simulink model "MOTOR_GENERATOR_SYSTEM_SIMULINK"  (R2023a)
settings: Solver=ode4  StartTime=0.0  StopTime=6.0  FixedStep=StepSize  RelTol=1e-3
values from neighbouring files (symbols this model uses):
  Jg = 0.05    [MOTOR_GENERATOR_SYSTEM_SCRIPT.m]
  Jm = 0.04    [MOTOR_GENERATOR_SYSTEM_SCRIPT.m]
  kag = 0.25    [MOTOR_GENERATOR_SYSTEM_SCRIPT.m]
  kam = 0.3    [MOTOR_GENERATOR_SYSTEM_SCRIPT.m]
  kfg = 0.0008    [MOTOR_GENERATOR_SYSTEM_SCRIPT.m]
  kfm = 0.0007    [MOTOR_GENERATOR_SYSTEM_SCRIPT.m]
  Lag = 0.06    [MOTOR_GENERATOR_SYSTEM_SCRIPT.m]
  Lam = 0.05    [MOTOR_GENERATOR_SYSTEM_SCRIPT.m]
  Rag = 0.3    [MOTOR_GENERATOR_SYSTEM_SCRIPT.m]
  Ram = 0.4    [MOTOR_GENERATOR_SYSTEM_SCRIPT.m]
settings Model: Creator=student  LastModifiedBy=student

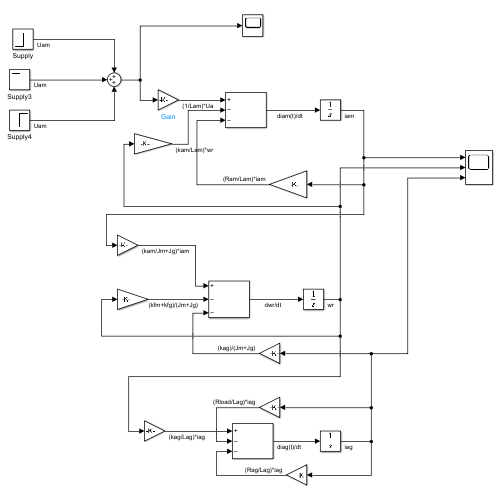
[thumbnail: Simulink's stored preview of the top-level diagram]
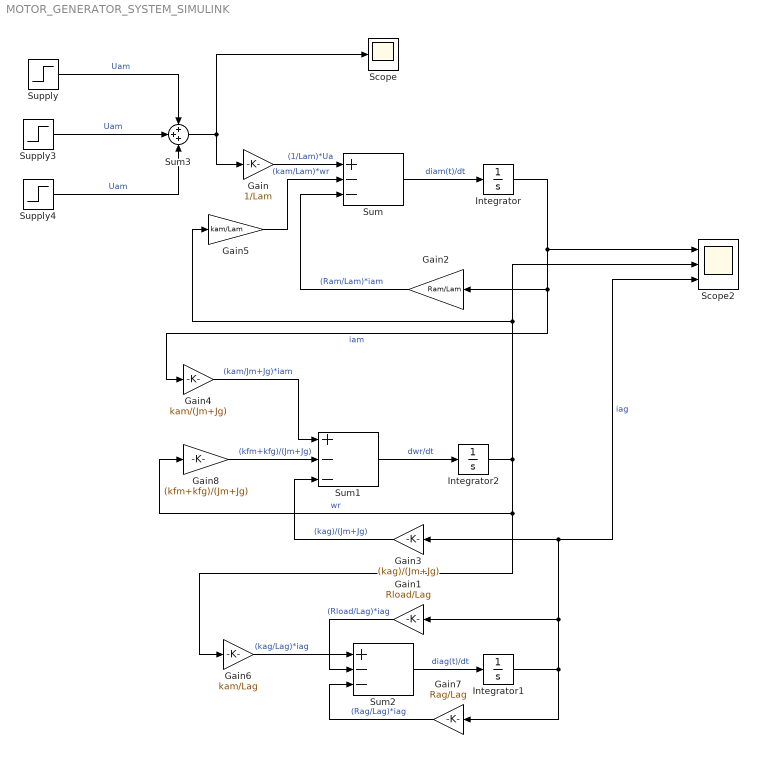
== system MOTOR_GENERATOR_SYSTEM_SIMULINK ==
  Gain : Gain  Gain=1/Lam
  Gain1 : Gain  Gain=Rload/Lag
  Gain2 : Gain  Gain=Ram/Lam
  Gain3 : Gain  Gain=(kag)/(Jm+Jg)
  Gain4 : Gain  Gain=kam/(Jm+Jg)
  Gain5 : Gain  Gain=kam/Lam
  Gain6 : Gain  Gain=kam/Lag
  Gain7 : Gain  Gain=Rag/Lag
  Gain8 : Gain  Gain=(kfm+kfg)/(Jm+Jg)
  Integrator : Integrator
  Integrator1 : Integrator
  Integrator2 : Integrator
  Scope : Scope
  Scope2 : Scope  NumInputPorts=3
  Sum : Sum  Inputs=+--
  Sum1 : Sum  Inputs=+--
  Sum2 : Sum  Inputs=+--
  Sum3 : Sum  Inputs=+++
  Supply : Step  Time=0  Before=100  After=100  SampleTime=0
  Supply3 : Step  Time=2  After=-50  SampleTime=0
  Supply4 : Step  Time=4  After=25  SampleTime=0
  wires:
  Gain5/1 -> Sum/2  "(kam/Lam)*wr"
  Gain/1 -> Sum/1  "(1/Lam)*Ua"
  Gain4/1 -> Sum1/1  "(kam/Jm+Jg)*iam"
  Sum/1 -> Integrator/1  "diam(t)/dt"
  Gain2/1 -> Sum/3  "(Ram/Lam)*iam"
  Integrator/1 -> Gain4/1, Gain2/1, Scope2/1  "iam"
  Integrator2/1 -> Gain8/1, Gain6/1, Scope2/2, Gain5/1  "wr"
  Sum1/1 -> Integrator2/1  "dwr/dt"
  Sum2/1 -> Integrator1/1  "diag(t)/dt"
  Gain1/1 -> Sum2/2  "(Rload/Lag)*iag"
  Integrator1/1 -> Gain7/1, Scope2/3, Gain3/1, Gain1/1  "iag"
  Gain6/1 -> Sum2/1  "(kag/Lag)*iag"
  Gain7/1 -> Sum2/3  "(Rag/Lag)*iag"
  Gain8/1 -> Sum1/2  "(kfm+kfg)/(Jm+Jg)"
  Gain3/1 -> Sum1/3  "(kag)/(Jm+Jg)"
  Supply/1 -> Sum3/1  "Uam"
  Supply3/1 -> Sum3/2  "Uam"
  Sum3/1 -> Scope/1, Gain/1
  Supply4/1 -> Sum3/3  "Uam"
